simulink model "Daolibai_jianmotu"  (R2020b)
settings: Solver=VariableStepAuto  StartTime=0.0  StopTime=50  MaxStep=1e-3  RelTol=1e-3
settings Model: Creator=19017  LastModifiedBy=19017
settings OptimizationCC: LifeSpan=inf
settings DebuggingCC: ArithmeticOperatorsInVariantConditions=warning
settings SFSimCC: CustomCodeUndefinedFunction=UseInterfaceOnly
settings CodeAppCC: StateflowObjectComments=on

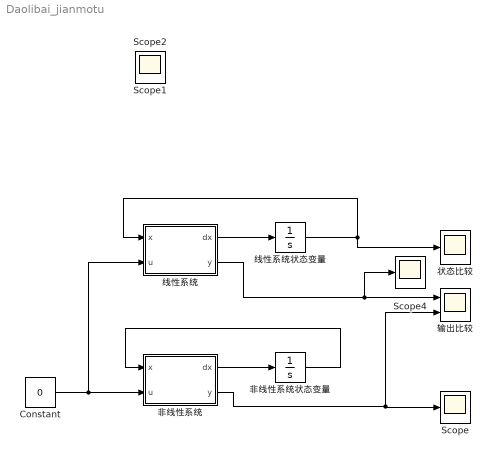
== system Daolibai_jianmotu ==
  Constant : Constant  Value=0
  Scope{,1..2,4} (4 alike) : Scope
  状态比较 : Scope
  线性系统 : MATLAB Function  TreatAsAtomicUnit=on
  线性系统状态变量 : Integrator  InitialCondition=[0 0 0.01 0]
  输出比较 : Scope  NumInputPorts=2
  非线性系统 : MATLAB Function  TreatAsAtomicUnit=on
  非线性系统状态变量 : Integrator  InitialCondition=[0 0 0.01 0]
  wires:
  非线性系统状态变量/1 -> 非线性系统/1(x)
  非线性系统/2(y) -> Scope/1, 输出比较/2
  非线性系统/1(dx) -> 非线性系统状态变量/1
  线性系统/1(dx) -> 线性系统状态变量/1
  线性系统状态变量/1 -> 线性系统/1(x), 状态比较/1
  Constant/1 -> 线性系统/2(u), 非线性系统/2(u)
  线性系统/2(y) -> Scope4/1, 输出比较/1

== matlab function Daolibai_jianmotu/非线性系统 ==
  data: dx output; x input; u input; y output
% function [dx,y] = fcn(x,u)
% M = 1;
% m = 0.1;
% l = 0.5;
% g = 9.8;
% x1=x(1);
% x2=x(2);
% x3=x(3);
% x4=x(4);
% 
% dx1 = x2;
% dx2 =(u + m*l*x4*x4*sin(x3) - m*g*sin(x3)*cos(x3))/(M + m - m*cos(x3)*cos(x3));
% dx3 = x4;
% dx4 =(-u*cos(x3) + (M+m)*g*sin(x3) - m*l*x4*x4*sin(x3)*cos(x3))/((M+m)*l - m*l*cos(x3)*cos(x3));
% dx = [dx1;dx2;dx3;dx4];
% y=x1;

function [dx,y] = fcn(x,u) %非线性系统模型
dx = zeros(4,1);%返回4x1的全0矩阵
M = 1;
m = 0.1;
l = 0.5;
g = 9.8;
dx(1) = x(2);
dx(2) = (u+m*l*x(4)^2*sin(x(3))-m*g*sin(x(3))*cos(x(3)))/(M+m-m*cos(x(3))^2);
dx(3) = x(4);
dx(4) = (-u*cos(x(3))+(M+m)*g*sin(x(3))-m*l*x(4)^2*sin(x(3))*cos(x(3)))/((M+m)*l-m*l*cos(x(3))^2);
y = x(1);

== matlab function Daolibai_jianmotu/线性系统 ==
  data: x input; dx output; u input; y output
function [dx,y] = fcn(x,u)%线性系统模型
dx = zeros(4,1);
M = 1;
m = 0.1;
l = 0.5;
g = 9.8;
dx(1) = x(2);
dx(2) = -m*g*x(3)/M+u/M;
dx(3) = x(4);
dx(4) = (M+m)*g*x(3)/(M*l)-u/(M*l);
y = x(1);
